simulink model "chap7_2sim"  (R2015a)
settings: Solver=ode45  StartTime=0.0  StopTime=10  FixedStep=0.01  RelTol=1e-3
settings Model: Creator=Masoud  LastModifiedBy=Masoud

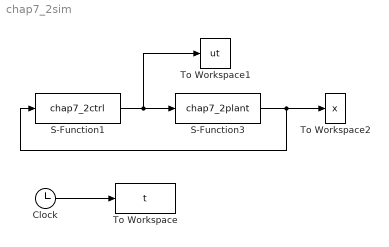
== system chap7_2sim ==
  Clock : Clock
  S-Function1 : S-Function  FunctionName=chap7_2ctrl  SFunctionModules='chap7_2ctrl'
  S-Function3 : S-Function  FunctionName=chap7_2plant  SFunctionModules='chap7_2plant'
  To Workspace : ToWorkspace  VariableName=t  SampleTime=-1
  To Workspace1 : ToWorkspace  VariableName=ut  SampleTime=-1
  To Workspace2 : ToWorkspace  VariableName=x  SampleTime=-1
  wires:
  Clock/1 -> To Workspace/1
  S-Function3/1 -> S-Function1/1, To Workspace2/1
  S-Function1/1 -> S-Function3/1, To Workspace1/1
